simulink model "Three_Phase_SPWM"  (Simulink 7.5)
settings: Solver=ode45  StartTime=0.0  StopTime=0.04  RelTol=1e-3
libraries: powerlib x8, powerlib_extras x4
settings Model: Creator=lm  LastModifiedBy=lm

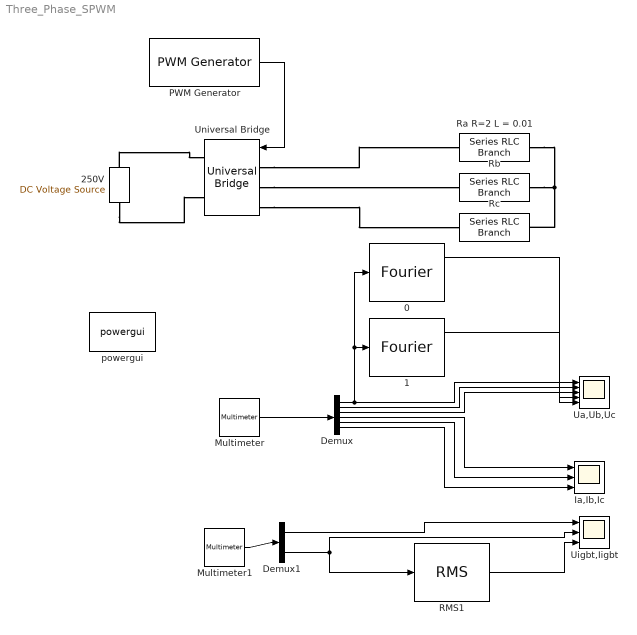
== system Three_Phase_SPWM ==
  0 : powerlib_extras/Measurements/Fourier  DialogController=POWERSYS.PowerSysDialog  SystemSampleTime=-1  f1=50  n=0
  1 : powerlib_extras/Measurements/Fourier  DialogController=POWERSYS.PowerSysDialog  SystemSampleTime=-1  f1=50  n=1
  250V : powerlib/Electrical Sources/DC Voltage Source  DialogController=POWERSYS.PowerSysDialog  SystemSampleTime=-1  Amplitude=250  Measurements=None
  Demux : Demux  Outputs=6
  Demux1 : Demux  Outputs=2
  Ia,Ib,Ic : Scope  NumInputPorts=3
      settings: YMin=-5~-5~-5  YMax=5~5~5
  Multimeter : powerlib/Measurements/Multimeter  SystemSampleTime=-1  PhasorSimulation=off  OutputType=Complex  sel=[1 2 3 14 15 16]  L=22  Gain=[1 1 1 1 1 1]  yselected={'Ub: Ra R=2 L = 0.01','Ub: Rb','Ub: Rc','Ib: Ra R=2 L = 0.01','Ib: Rb','Ib: Rc'};  PSBOutputType=1  PSBequivalent=0  AxesSetting=[0,0.1,-100,100]  Display=0  SavedBlockNames=-11
  Multimeter1 : powerlib/Measurements/Multimeter  SystemSampleTime=-1  PhasorSimulation=off  OutputType=Complex  sel=[4 17]  L=22  Gain=[1 1]  yselected={'Usw1: Universal Bridge','Isw1: Universal Bridge'};  PSBOutputType=1  PSBequivalent=0  AxesSetting=[0,0.1,-100,100]  Display=0  SavedBlockNames=-11
  PWM Generator : powerlib_extras/Control  Blocks/PWM Generator  DialogController=POWERSYS.PowerSysDialog  SystemSampleTime=-1  GeneratorMode="3-arm  bridge (6 pulses)"  Fc=600  Internal=on  mIndex=0.8  Freq=50  Phase=0
  RMS1 : powerlib_extras/Measurements/RMS  DialogController=POWERSYS.PowerSysDialog  SystemSampleTime=-1  f1=50
  Ra R=2 L = 0.01 : powerlib/Elements/Series RLC Branch  DialogController=POWERSYS.PowerSysDialog  PhysicalDomain=powersysdomain  SubClassName=unknown  LeftPortType=p1  RightPortType=p1  LConnTagsString=__new0  RConnTagsString=__new0  BranchType=RL  Resistance=2  Inductance=1e-2  SetiL0=off  InitialCurrent=0  Capacitance=1e-6  Setx0=off  InitialVoltage=0  Measurements=Branch voltage and current
  Rb : powerlib/Elements/Series RLC Branch  DialogController=POWERSYS.PowerSysDialog  PhysicalDomain=powersysdomain  SubClassName=unknown  LeftPortType=p1  RightPortType=p1  LConnTagsString=__new0  RConnTagsString=__new0  BranchType=RL  Resistance=2  Inductance=1e-2  SetiL0=off  InitialCurrent=0  Capacitance=1e-6  Setx0=off  InitialVoltage=0  Measurements=Branch voltage and current
  Rc : powerlib/Elements/Series RLC Branch  DialogController=POWERSYS.PowerSysDialog  PhysicalDomain=powersysdomain  SubClassName=unknown  LeftPortType=p1  RightPortType=p1  LConnTagsString=__new0  RConnTagsString=__new0  BranchType=RL  Resistance=2  Inductance=1e-2  SetiL0=off  InitialCurrent=0  Capacitance=1e-6  Setx0=off  InitialVoltage=0  Measurements=Branch voltage and current
  Ua,Ub,Uc : Scope  NumInputPorts=5
      settings: YMin=-5~-5~-5~-5~-5  YMax=5~5~5~5~5
  Uigbt,Iigbt : Scope  NumInputPorts=3
      settings: YMin=-5~-5~-5  YMax=5~5~5  SaveName=ScopeData2
  Universal Bridge : powerlib/Power Electronics/Universal Bridge  DialogController=POWERSYS.PowerSysDialog  SystemSampleTime=-1  Arms=3  SnubberResistance=1e3  SnubberCapacitance=1e-6  Device=IGBT / Diodes  Ron=1e-4  Lon=0  ForwardVoltages="[  0  0  ]"  ForwardVoltage=0  GTOparameters=[ 10e-6 , 20e-6 ]  IGBTparameters=[ 1e-6 , 0 ]  Measurements=All voltages and currents  Measurements_2=None  converterType=Rectifier
  powergui : powerlib/powergui  Priority=1  SystemSampleTime=-1  SimulationMode=Discrete  SampleTime=50e-6  frequency=60  SPID=off  DisableSnubberDevices=off  DisableRonSwitches=off  DisableVfSwitches=off  SwTol=0  Interpol=off  frequencyindice=0  echomessages=off  HookPort=off  DisplayEquations=off  FunctionMessages=off  EnableUseOfTLC=off  x0status=blocks  RestoreLinks=warning  ResistiveCurrentMeasurement=off  Ylog=off  Xlog=on  ShowGrid=off  save=off  variable=ZData  ZoomFFT=off  StartTime=0.0  cycles=1  DisplayStyle=1  FreqAxis=off  MaxFrequency=1000  frequencyindicesteady=1  display=off  methode=off
  wires:
  PWM Generator/1 -> Universal Bridge/1
  Multimeter/1 -> Demux/1
  Demux/4 -> Ia,Ib,Ic/1
  Demux/5 -> Ia,Ib,Ic/2
  Demux/6 -> Ia,Ib,Ic/3
  Demux/1 -> Ua,Ub,Uc/1, 0/1, 1/1
  Demux/2 -> Ua,Ub,Uc/2
  Demux/3 -> Ua,Ub,Uc/3
  0/1 -> Ua,Ub,Uc/4
  1/1 -> Ua,Ub,Uc/5
  Multimeter1/1 -> Demux1/1
  Demux1/1 -> Uigbt,Iigbt/1
  Demux1/2 -> Uigbt,Iigbt/2, RMS1/1
  RMS1/1 -> Uigbt,Iigbt/3
  connections:
  250V/RConn1 -- Universal Bridge/RConn1
  250V/LConn1 -- Universal Bridge/RConn2
  Universal Bridge/LConn1 -- Ra R=2 L = 0.01/LConn1
  Universal Bridge/LConn2 -- Rb/LConn1
  Universal Bridge/LConn3 -- Rc/LConn1
  Ra R=2 L = 0.01/RConn1 -- Rc/RConn1 -- Rb/RConn1
